simulink model "TuneControllers"  (R2020b)
settings: Solver=VariableStepAuto  StartTime=0.0  StopTime=10  RelTol=1e-3
undefined symbols (not defined in the file): Controller_Mode, DiscIntNeverNeededParam, Tests_Enum_SpectralTestSystem, ts_control
libraries: simulink x4
settings Model: DataDictionary=Dictionary.sldd  EnableAccessToBaseWorkspace=off  OrderedModelArguments=off  Creator=alons  LastModifiedBy=alons

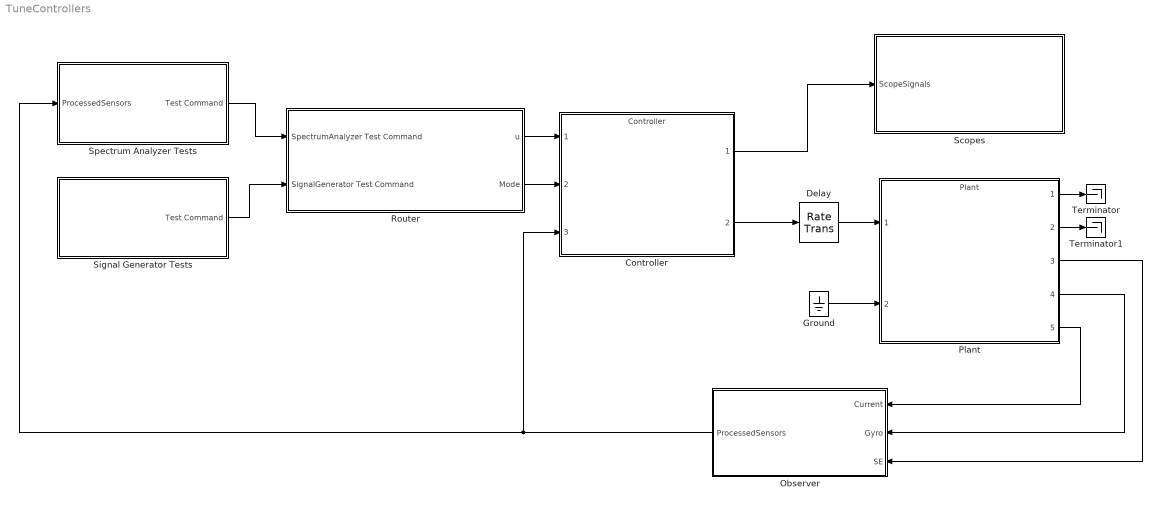
== system TuneControllers ==
  Controller : ModelReference  ModelNameDialog=Controller  SimulationMode=Normal  ModelReferenceVersion=1.79
  Delay : RateTransition  OutPortSampleTime=0
  Ground : Ground
  Observer : Subsystem  TreatAsAtomicUnit=on
  Plant : ModelReference  ModelNameDialog=Plant.slx  SimulationMode=Normal  ModelReferenceVersion=1.81  SimulationMode=Normal
  Router : Subsystem  TreatAsAtomicUnit=on
  Scopes : Subsystem
  Signal Generator Tests : Subsystem  TreatAsAtomicUnit=on
  Spectrum Analyzer Tests : Subsystem  TreatAsAtomicUnit=on
  Terminator : Terminator
  Terminator1 : Terminator
  wires:
  Delay/1 -> Plant/1
  Ground/1 -> Plant/2
  Observer/1(ProcessedSensors) -> Controller/3, Spectrum Analyzer Tests/1(ProcessedSensors)
  Signal Generator Tests/1(Test Command) -> Router/2(SignalGenerator Test Command)
  Spectrum Analyzer Tests/1(Test Command) -> Router/1(SpectrumAnalyzer Test Command)
  Router/1(u) -> Controller/1
  Router/2(Mode) -> Controller/2
  Plant/1 -> Terminator/1
  Controller/2 -> Delay/1
  Plant/5 -> Observer/1(Current)
  Plant/4 -> Observer/2(Gyro)
  Plant/3 -> Observer/3(SE)
  Plant/2 -> Terminator1/1
  Controller/1 -> Scopes/1(ScopeSignals)

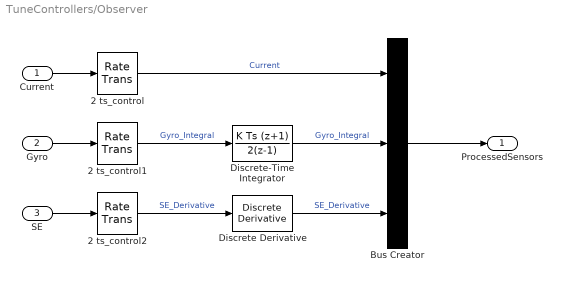
== system TuneControllers/Observer ==
  Current : Inport  SampleTime=ts_control
  Gyro : Inport  Port=2  SampleTime=ts_control
  SE : Inport  Port=3  SampleTime=ts_control
  2 ts_control : RateTransition  OutPortSampleTime=ts_control
  2 ts_control1 : RateTransition  OutPortSampleTime=ts_control
  2 ts_control2 : RateTransition  OutPortSampleTime=ts_control
  Bus Creator : BusCreator  Inputs=3  OutDataTypeStr=Bus: Processed_Sensors
  Discrete Derivative : simulink/Discrete/Discrete Derivative  gainval=1.0  ICPrevScaledInput=0.0  OutMin=[]  OutMax=[]  OutDataType=fixdt(1, 16)  OutScaling=2^-10  DoSatur=off
  Discrete-Time Integrator : DiscreteIntegrator  IntegratorMethod=Integration: Trapezoidal  SampleTime=-1  ICPrevOutput=DiscIntNeverNeededParam  ICPrevScaledInput=DiscIntNeverNeededParam
  ProcessedSensors : Outport  OutDataTypeStr=Bus: Processed_Sensors  SampleTime=ts_control
  wires:
  Bus Creator/1 -> ProcessedSensors/1
  Discrete Derivative/1 -> Bus Creator/3  "SE_Derivative"
  Discrete-Time Integrator/1 -> Bus Creator/2  "Gyro_Integral"
  2 ts_control1/1 -> Discrete-Time Integrator/1  "Gyro_Integral"
  Gyro/1 -> 2 ts_control1/1
  2 ts_control2/1 -> Discrete Derivative/1  "SE_Derivative"
  SE/1 -> 2 ts_control2/1
  Current/1 -> 2 ts_control/1
  2 ts_control/1 -> Bus Creator/1  "Current"

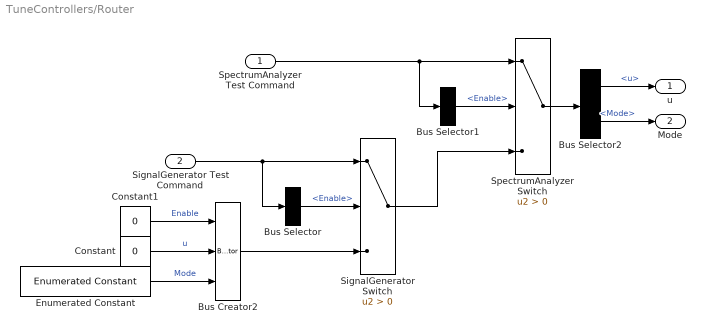
== system TuneControllers/Router ==
  SpectrumAnalyzer Test Command : Inport
  SignalGenerator Test Command : Inport  Port=2
  Bus Creator2 : BusCreator  Inputs=3
  Bus Selector : BusSelector  OutputSignals=Enable
  Bus Selector1 : BusSelector  OutputSignals=Enable
  Bus Selector2 : BusSelector  OutputSignals=u,Mode
  Constant : Constant  Value=0
  Constant1 : Constant  Value=0
  Enumerated Constant : simulink/Sources/Enumerated Constant  OutDataTypeStr=Enum: Controller_Mode  Value=Controller_Mode.Voltage  SampleTime=inf
  SignalGenerator Switch : Switch  Criteria=u2 > Threshold
  SpectrumAnalyzer Switch : Switch  Criteria=u2 > Threshold
  u : Outport
  Mode : Outport  Port=2
  wires:
  SignalGenerator Test Command/1 -> Bus Selector/1, SignalGenerator Switch/1
  Enumerated Constant/1 -> Bus Creator2/3  "Mode"
  Constant/1 -> Bus Creator2/2  "u"
  Bus Creator2/1 -> SignalGenerator Switch/3
  Bus Selector/1 -> SignalGenerator Switch/2  "<Enable>"
  SpectrumAnalyzer Test Command/1 -> Bus Selector1/1, SpectrumAnalyzer Switch/1
  Bus Selector1/1 -> SpectrumAnalyzer Switch/2  "<Enable>"
  SignalGenerator Switch/1 -> SpectrumAnalyzer Switch/3
  SpectrumAnalyzer Switch/1 -> Bus Selector2/1
  Constant1/1 -> Bus Creator2/1  "Enable"
  Bus Selector2/1 -> u/1  "<u>"
  Bus Selector2/2 -> Mode/1  "<Mode>"

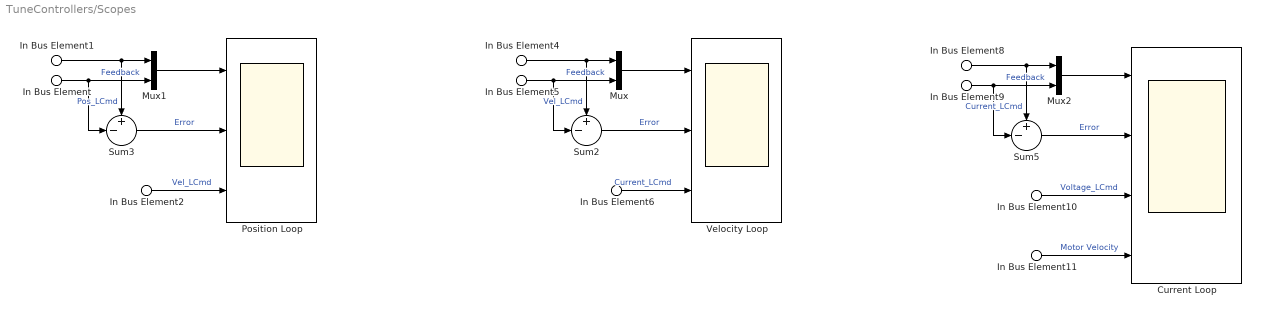
== system TuneControllers/Scopes ==
  In Bus Element : Inport  PortName=ScopeSignals  Element=Position.Gyro_Integral
  In Bus Element1 : Inport  PortName=ScopeSignals  Element=Position.Pos_LCmd
  In Bus Element2 : Inport  PortName=ScopeSignals  Element=Position.Vel_LCmd
  In Bus Element4 : Inport  PortName=ScopeSignals  Element=Velocity.Vel_LCmd
  In Bus Element5 : Inport  PortName=ScopeSignals  Element=Velocity.SE_Derivative
  In Bus Element6 : Inport  PortName=ScopeSignals  Element=Velocity.Current_LCmd
  In Bus Element8 : Inport  PortName=ScopeSignals  Element=Current.Current_LCmd
  In Bus Element9 : Inport  PortName=ScopeSignals  Element=Current.Current
  In Bus Element10 : Inport  PortName=ScopeSignals  Element=Current.Voltage_LCmd
  In Bus Element11 : Inport  PortName=ScopeSignals  Element=Current.SE_Derivative
  Current Loop : Scope  NumInputPorts=4
  Mux : Mux  Inputs=2
  Mux1 : Mux  Inputs=2
  Mux2 : Mux  Inputs=2
  Position Loop : Scope  NumInputPorts=3
  Sum2 : Sum  Inputs=+-|
  Sum3 : Sum  Inputs=+-|
  Sum5 : Sum  Inputs=+-|
  Velocity Loop : Scope  NumInputPorts=3
  wires:
  In Bus Element/1 -> Sum3/2, Mux1/2  "Feedback"
  In Bus Element8/1 -> Sum5/1, Mux2/1  "Current_LCmd"
  Sum5/1 -> Current Loop/2  "Error"
  In Bus Element10/1 -> Current Loop/3  "Voltage_LCmd"
  In Bus Element2/1 -> Position Loop/3  "Vel_LCmd"
  Mux2/1 -> Current Loop/1
  In Bus Element9/1 -> Sum5/2, Mux2/2  "Feedback"
  In Bus Element11/1 -> Current Loop/4  "Motor Velocity"
  In Bus Element5/1 -> Sum2/2, Mux/2  "Feedback"
  In Bus Element1/1 -> Sum3/1, Mux1/1  "Pos_LCmd"
  Mux/1 -> Velocity Loop/1
  In Bus Element6/1 -> Velocity Loop/3  "Current_LCmd"
  Mux1/1 -> Position Loop/1
  Sum3/1 -> Position Loop/2  "Error"
  In Bus Element4/1 -> Sum2/1, Mux/1  "Vel_LCmd"
  Sum2/1 -> Velocity Loop/2  "Error"

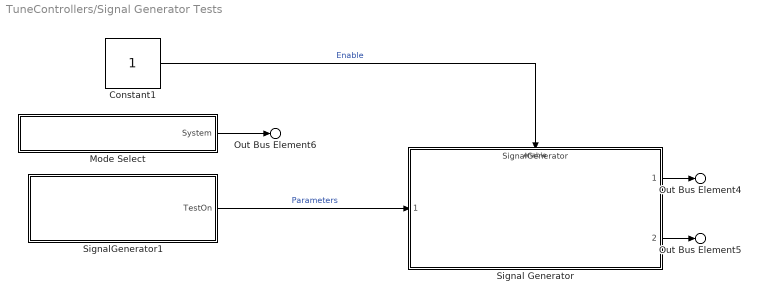
== system TuneControllers/Signal Generator Tests ==
  Constant1 : Constant  OutDataTypeStr=boolean
      settings: OpenFcn=|
      | if get_param(gcbh,'value')-48 set_param(gcbh,'value','0','backgroundcolor','red');
      | else set_param(gcbh,'value','1','backgroundcolor','green');
      | end
  Mode Select : Subsystem  mask(System Select){AxisMode=Velocity}
      mask prompts: AxisMode "Axis Mode for Test:"
      mask help: Specify the axis for test
      mask TypeOptions AxisMode: Voltage | Current | Velocity | Position
      mask Display:
      | Message = ['Selected Axis Mode: \n ' get_param(gcb,'AxisMode')];
      | disp(Message);
  Signal Generator : ModelReference  ModelNameDialog=SignalGenerator.slx  SimulationMode=Normal  ModelReferenceVersion=1.33  EnablePortName=Enable  EnablePortStatesWhenEnabling=reset
  SignalGenerator1 : Subsystem  mask(Signal Generator Parameters){TestType=Square wave, PeriodTime=2, Amplitude=20*pi/180, Bias=0, PulseWidth=20, NumberOfPeriods=100, ConstValue=1*pi/180}
      mask prompts: PeriodTime "Period time"; PulseWidth "Pulse width (%)"; NumberOfPeriods "Number of periods"
      mask help:
      | Comfy mask to create the input bus for Signal Generator.
      | If Constant is selected, only the ConstVal field is relevant.
      | (c) Alon Spinner 2021
      mask TypeOptions TestType: Square wave through zero | Square wave | Sine | Triangle | Pulse | Constant
      mask Callback TestType:
      | MaskObj=Simulink.Mask.get(gcb);
      | PeriodTimeObj= MaskObj.getParameter('PeriodTime');
      | AmplitudeObj= MaskObj.getParameter('Amplitude');
      | BiasObj= MaskObj.getParameter('Bias');
      | PulseWidthObj= MaskObj.getParameter('PulseWidth');
      | NumberOfPeriodsObj= MaskObj.getParameter('NumberOfPeriods');
      | ConstValueObj= MaskObj.getParameter('ConstValue');
      | 
      | switch get_param(gcb,'TestType')
      | 
      |     case {'Square wave through zero','Square wave','Sine','Triangle'}
      |         PeriodTimeObj.Visible='on';
      |         AmplitudeObj.Visible='on';
      |         BiasObj.Visible='on';
      |         PulseWidthObj.Visible='off';
      |         NumberOfPeriodsObj.Visible='on';
      |         ConstValueObj.Visible='off';
      |     case 'Pulse'
      |         PeriodTimeObj.Visible='on';
      |         AmplitudeObj.Visible='on';
      |         BiasObj.Visible='on';
      |         PulseWidthObj.Visible='on';
      |         NumberOfPeriodsObj.Visible='on';
      |         ConstValueObj.Visible='off';
      |     case 'Constant'
      |         PeriodTimeObj.Visible='off';
      |         AmplitudeObj.Visible='off';
      |         BiasObj.Visible='off';
      |         PulseWidthObj.Visible='off';
      |         NumberOfPeriodsObj.Visible='off';
      |         ConstValueObj.Visible='on';
      | end
      mask Display:
      | disp('Signal Generator Parameters\n----------------------------\n\n\n\n')
      | 
      | switch TestType
      |     case 1
      |         disp('\n\nTest Type:\nSquare wave through zero')
      |     case 2
      |         disp('\n\nTest Type:\nSquare wave')
      |     case 3
      |         disp('\n\nTest Type:\nSine wave')
      |     case 4
      |         disp('\n\nTest Type:\nTriangle wave')
      |     case 5
      |         disp('\n\nTest Type:\nPulse')
      |     case 6
      |         disp('\n\nTest Type:\nConstant')
      | end
  Out Bus Element4 : Outport  PortName=Test Command  Element=Enable
  Out Bus Element5 : Outport  PortName=Test Command  Element=u
  Out Bus Element6 : Outport  PortName=Test Command  Element=Mode
  wires:
  Constant1/1 -> Signal Generator/Enable  "Enable"
  SignalGenerator1/1(TestOn) -> Signal Generator/1  "Parameters"
  Mode Select/1(System) -> Out Bus Element6/1
  Signal Generator/2 -> Out Bus Element5/1
  Signal Generator/1 -> Out Bus Element4/1

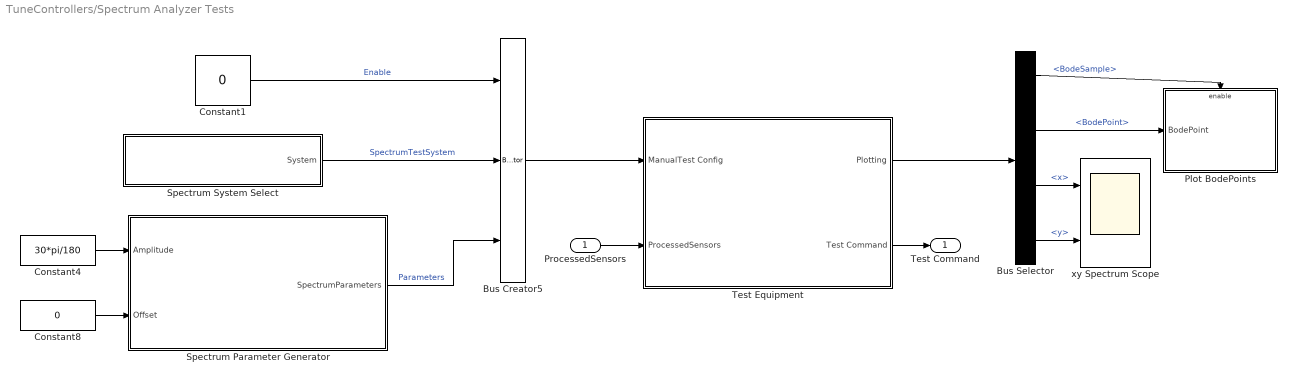
== system TuneControllers/Spectrum Analyzer Tests ==
  ProcessedSensors : Inport
  Bus Creator5 : BusCreator  Inputs=3
  Bus Selector : BusSelector  OutputSignals=BodeSample,BodePoint,x,y
  Constant1 : Constant  Value=0  OutDataTypeStr=boolean
      settings: OpenFcn=|
      | if get_param(gcbh,'value')-48 set_param(gcbh,'value','0','backgroundcolor','red');
      | else set_param(gcbh,'value','1','backgroundcolor','green');
      | end
  Constant4 : Constant  Value=30*pi/180  OutDataTypeStr=Inherit: Inherit via back propagation
  Constant8 : Constant  Value=0  OutDataTypeStr=Inherit: Inherit via back propagation
  Plot BodePoints : Subsystem
  Spectrum Parameter Generator : Subsystem  mask{PhaseIn=0, Start_Frequency=1, Stop_Frequency=500, Min_PeriodsPerSine=5, Min_PointsPerSine=150, LinearOrLog=Logarithmic, Linear_Step_Frequency=0.1, Logarithmic_NumOfPoints=250, OLCL=CL}
      mask prompts: PhaseIn "Phase In [rad]"; Start_Frequency "Start Frequency [Hz]"; Stop_Frequency "Stop Frequency [Hz]"; Min_PeriodsPerSine "Minimal Number of periods per frequency"; Min_PointsPerSine "Minimal Number of sampled points per frequency"; LinearOrLog "Frequency axis type"; Linear_Step_Frequency "Step Frequency [Hz] (for linear test type)"; Logarithmic_NumOfPoints "Number of points (for logarithmic test type)"; OLCL "Measurement Type"
      mask init:
      | switch LinearOrLog
      |     case 1
      |         f = Start_Frequency:Linear_Step_Frequency:Stop_Frequency;
      |         n = length(f);
      |     case 2
      |         n = 1:Logarithmic_NumOfPoints;
      |         f = 10.^((log10(Stop_Frequency) - log10(Start_Frequency))/Logarithmic_NumOfPoints*n + log10(Start_Frequency));
      | end
      | %%%%%%%%%%%%%%%%%%%%%%%%%%%%
      | ts=1/1024; %assumption
      | T_min=Min_PointsPerSine*ts; %scalar
      | T_minPeriodsPerSine=Min_PeriodsPerSine*(1./f); %vector
      | T=sum(max(T_minPeriodsPerSine,T_min));
      | 
      | y = T/60; 
      | h = floor(y/60); %[hours]
      | m = floor(((y/60)-h)*60); %[min]
      | s = round((y-floor(y))*60); %[sec]
      mask TypeOptions LinearOrLog: Linear | Logarithmic
      mask Callback LinearOrLog:
      | MaskObj = Simulink.Mask.get(gcb);
      | Linear_Step_Frequency_Obj= MaskObj.getParameter('Linear_Step_Frequency');
      | Logarithmic_NumOfPoints_Obj= MaskObj.getParameter('Logarithmic_NumOfPoints');
      | 
      | LinearOrLog = get_param(gcb,'LinearOrLog');
      | switch LinearOrLog
      |     case 'Linear'
      |     Linear_Step_Frequency_Obj.Visible='on';
      |     Logarithmic_NumOfPoints_Obj.Visible='off';
      |     case 'Logarithmic'
      |     Linear_Step_Frequency_Obj.Visible='off';
      |     Logarithmic_NumOfPoints_Obj.Visible='on';
      | end
      mask TypeOptions OLCL: OL | CL
      mask DialogControl Container3 Prompt: Test Type
      mask Display:
      | str = sprintf(['-----------------\n'...
      |     'SPECTRUM\nParameter\nGenerator\n',...
      |     '------------------\n',...
      |     'Estimated test time:\n',...
      |     '%02d:%02d:%02d\n[hh:mm:ss]'],h,m,s);
      | disp(str)
  Spectrum System Select : Subsystem  mask(System Select){SpectralTestSystem=SE_Velocity_CL}
      mask help: Specify the axis for test
      mask TypeOptions SpectralTestSystem: NoSpectralTest | Current_Plant | Current_CL | SE_Velocity_Plant | SE_Velocity_CL | Gyro_Position_Plant | Gyro_Position_CL
      mask Display:
      | if ~strcmpi(get_param(gcb,'SpectralTestSystem'),'NoSpectralTest'),
      |     set_param(gcb,'BackgroundColor','Green');
      |     Message = [' *** ACTIVE *** \n Selected Axis: \n ' get_param(gcb,'SpectralTestSystem')];
      | else
      |     set_param(gcb,'BackgroundColor','Red');
      |      Message = [' *** deactivated ***'];
      | end
      | 
      | disp(Message);
  Test Equipment : Subsystem  TreatAsAtomicUnit=on
  xy Spectrum Scope : Scope  NumInputPorts=2
  Test Command : Outport
  wires:
  Test Equipment/2(Test Command) -> Test Command/1
  Bus Creator5/1 -> Test Equipment/1(ManualTest Config)
  Constant1/1 -> Bus Creator5/1  "Enable"
  Constant4/1 -> Spectrum Parameter Generator/1(Amplitude)
  Constant8/1 -> Spectrum Parameter Generator/2(Offset)
  Spectrum System Select/1(System) -> Bus Creator5/2  "SpectrumTestSystem"
  Bus Selector/3 -> xy Spectrum Scope/1  "<x>"
  Bus Selector/1 -> Plot BodePoints/Enable  "<BodeSample>"
  Bus Selector/2 -> Plot BodePoints/1(BodePoint)  "<BodePoint>"
  Bus Selector/4 -> xy Spectrum Scope/2  "<y>"
  Test Equipment/1(Plotting) -> Bus Selector/1
  Spectrum Parameter Generator/1(SpectrumParameters) -> Bus Creator5/3  "Parameters"
  ProcessedSensors/1 -> Test Equipment/2(ProcessedSensors)

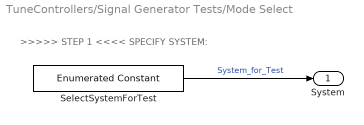
== system TuneControllers/Signal Generator Tests/Mode Select ==
  note: >>>>> STEP 1 <<<< SPECIFY SYSTEM:
  SelectSystemForTest : simulink/Sources/Enumerated Constant  OutDataTypeStr=Enum: Controller_Mode  Value=Controller_Mode(AxisMode)  SampleTime=inf
  System : Outport
  wires:
  SelectSystemForTest/1 -> System/1  "System_for_Test"

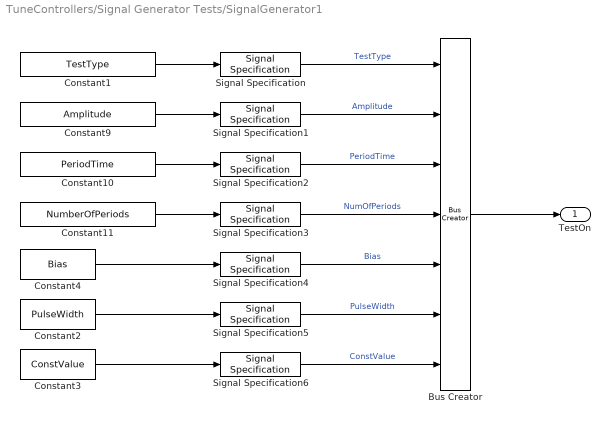
== system TuneControllers/Signal Generator Tests/SignalGenerator1 ==
  Bus Creator : BusCreator  Inputs=7  OutDataTypeStr=Bus: Tests_SignalGenerator_Parameters  NonVirtualBus=on
  Constant1 : Constant  Value=TestType  OutDataTypeStr=Inherit: Inherit via back propagation
  Constant10 : Constant  Value=PeriodTime  OutDataTypeStr=Inherit: Inherit via back propagation
  Constant11 : Constant  Value=NumberOfPeriods  OutDataTypeStr=Inherit: Inherit via back propagation
  Constant2 : Constant  Value=PulseWidth  OutDataTypeStr=Inherit: Inherit via back propagation
  Constant3 : Constant  Value=ConstValue  OutDataTypeStr=Inherit: Inherit via back propagation
  Constant4 : Constant  Value=Bias  OutDataTypeStr=Inherit: Inherit via back propagation
  Constant9 : Constant  Value=Amplitude  OutDataTypeStr=Inherit: Inherit via back propagation
  Signal Specification : SignalSpecification  OutDataTypeStr=int8
  Signal Specification{1..6} (6 alike) : SignalSpecification  OutDataTypeStr=double
  TestOn : Outport  OutDataTypeStr=Bus: Tests_SignalGenerator_Parameters  OutputWhenDisabled=reset  InitialOutput=0
  wires:
  Constant1/1 -> Signal Specification/1
  Constant9/1 -> Signal Specification1/1
  Constant4/1 -> Signal Specification4/1
  Constant11/1 -> Signal Specification3/1
  Constant10/1 -> Signal Specification2/1
  Bus Creator/1 -> TestOn/1
  Constant2/1 -> Signal Specification5/1
  Signal Specification/1 -> Bus Creator/1  "TestType"
  Signal Specification1/1 -> Bus Creator/2  "Amplitude"
  Signal Specification2/1 -> Bus Creator/3  "PeriodTime"
  Signal Specification3/1 -> Bus Creator/4  "NumOfPeriods"
  Signal Specification4/1 -> Bus Creator/5  "Bias"
  Signal Specification5/1 -> Bus Creator/6  "PulseWidth"
  Signal Specification6/1 -> Bus Creator/7  "ConstValue"
  Constant3/1 -> Signal Specification6/1

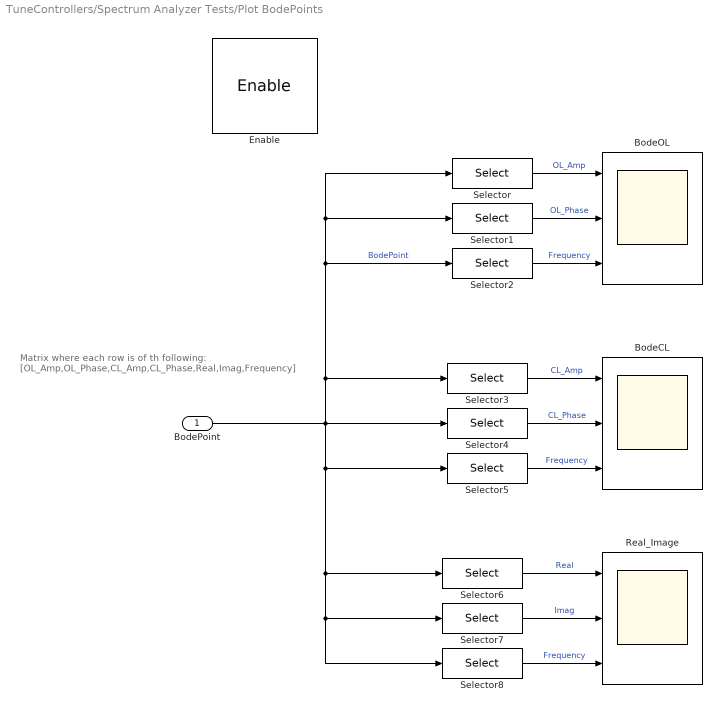
== system TuneControllers/Spectrum Analyzer Tests/Plot BodePoints ==
  note: Matrix where each row is of th following:
      | [OL_Amp,OL_Phase,CL_Amp,CL_Phase,Real,Imag,Frequency]
  BodePoint : Inport
  Enable : EnablePort  StatesWhenEnabling=reset
  BodeCL : Scope  NumInputPorts=3
  BodeOL : Scope  NumInputPorts=3
  Real_Image : Scope  NumInputPorts=3
  Selector : Selector  NumberOfDimensions=2  InputPortWidth=3  IndexOptions=Select all,Index vector (dialog)  Indices=1,1  OutputSizes=1,1
  Selector1 : Selector  NumberOfDimensions=2  InputPortWidth=3  IndexOptions=Select all,Index vector (dialog)  Indices=1,2  OutputSizes=1,1
  Selector2 : Selector  NumberOfDimensions=2  InputPortWidth=3  IndexOptions=Select all,Index vector (dialog)  Indices=1,7  OutputSizes=1,1
  Selector3 : Selector  NumberOfDimensions=2  InputPortWidth=3  IndexOptions=Select all,Index vector (dialog)  Indices=1,3  OutputSizes=1,1
  Selector4 : Selector  NumberOfDimensions=2  InputPortWidth=3  IndexOptions=Select all,Index vector (dialog)  Indices=1,4  OutputSizes=1,1
  Selector5 : Selector  NumberOfDimensions=2  InputPortWidth=3  IndexOptions=Select all,Index vector (dialog)  Indices=1,7  OutputSizes=1,1
  Selector6 : Selector  NumberOfDimensions=2  InputPortWidth=3  IndexOptions=Select all,Index vector (dialog)  Indices=1,5  OutputSizes=1,1
  Selector7 : Selector  NumberOfDimensions=2  InputPortWidth=3  IndexOptions=Select all,Index vector (dialog)  Indices=1,6  OutputSizes=1,1
  Selector8 : Selector  NumberOfDimensions=2  InputPortWidth=3  IndexOptions=Select all,Index vector (dialog)  Indices=1,7  OutputSizes=1,1
  wires:
  BodePoint/1 -> Selector/1, Selector1/1, Selector2/1, Selector3/1, Selector4/1, Selector5/1, Selector6/1, Selector7/1, Selector8/1  "BodePoint"
  Selector8/1 -> Real_Image/3  "Frequency"
  Selector7/1 -> Real_Image/2  "Imag"
  Selector6/1 -> Real_Image/1  "Real"
  Selector5/1 -> BodeCL/3  "Frequency"
  Selector4/1 -> BodeCL/2  "CL_Phase"
  Selector3/1 -> BodeCL/1  "CL_Amp"
  Selector2/1 -> BodeOL/3  "Frequency"
  Selector1/1 -> BodeOL/2  "OL_Phase"
  Selector/1 -> BodeOL/1  "OL_Amp"

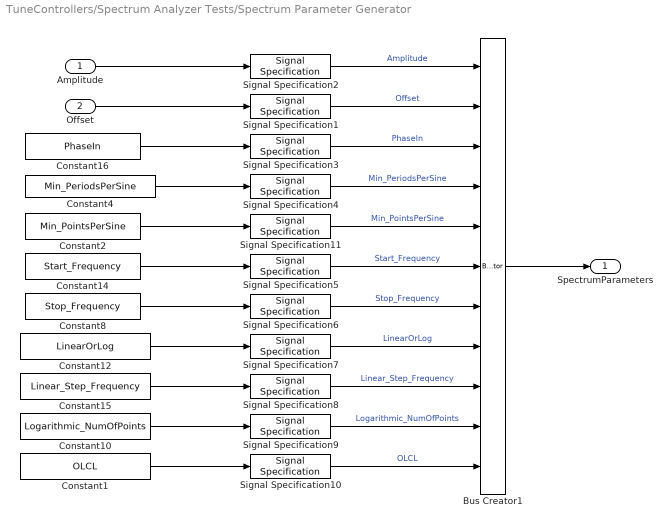
== system TuneControllers/Spectrum Analyzer Tests/Spectrum Parameter Generator ==
  Amplitude : Inport
  Offset : Inport  Port=2
  Bus Creator1 : BusCreator  Inputs=11  OutDataTypeStr=Bus: Tests_SpectrumAnalyzer_Parameters  NonVirtualBus=on
  Constant1 : Constant  Value=OLCL  OutDataTypeStr=Inherit: Inherit via back propagation
  Constant10 : Constant  Value=Logarithmic_NumOfPoints  OutDataTypeStr=Inherit: Inherit via back propagation
  Constant12 : Constant  Value=LinearOrLog  OutDataTypeStr=Inherit: Inherit via back propagation
  Constant14 : Constant  Value=Start_Frequency  OutDataTypeStr=Inherit: Inherit via back propagation
  Constant15 : Constant  Value=Linear_Step_Frequency  OutDataTypeStr=Inherit: Inherit via back propagation
  Constant16 : Constant  Value=PhaseIn  OutDataTypeStr=Inherit: Inherit via back propagation
  Constant2 : Constant  Value=Min_PointsPerSine  OutDataTypeStr=Inherit: Inherit via back propagation
  Constant4 : Constant  Value=Min_PeriodsPerSine  OutDataTypeStr=Inherit: Inherit via back propagation
  Constant8 : Constant  Value=Stop_Frequency  OutDataTypeStr=Inherit: Inherit via back propagation
  Signal Specification{1..6,8..9,11} (9 alike) : SignalSpecification  OutDataTypeStr=double
  Signal Specification10 : SignalSpecification  OutDataTypeStr=int8
  Signal Specification7 : SignalSpecification  OutDataTypeStr=int8
  SpectrumParameters : Outport  OutDataTypeStr=Bus: Tests_SpectrumAnalyzer_Parameters
  wires:
  Signal Specification11/1 -> Bus Creator1/5  "Min_PointsPerSine"
  Constant2/1 -> Signal Specification11/1
  Constant10/1 -> Signal Specification9/1
  Constant14/1 -> Signal Specification5/1
  Constant8/1 -> Signal Specification6/1
  Constant15/1 -> Signal Specification8/1
  Offset/1 -> Signal Specification1/1
  Amplitude/1 -> Signal Specification2/1
  Constant16/1 -> Signal Specification3/1
  Constant4/1 -> Signal Specification4/1
  Signal Specification2/1 -> Bus Creator1/1  "Amplitude"
  Signal Specification1/1 -> Bus Creator1/2  "Offset"
  Bus Creator1/1 -> SpectrumParameters/1
  Constant1/1 -> Signal Specification10/1
  Constant12/1 -> Signal Specification7/1
  Signal Specification3/1 -> Bus Creator1/3  "PhaseIn"
  Signal Specification4/1 -> Bus Creator1/4  "Min_PeriodsPerSine"
  Signal Specification5/1 -> Bus Creator1/6  "Start_Frequency"
  Signal Specification6/1 -> Bus Creator1/7  "Stop_Frequency"
  Signal Specification7/1 -> Bus Creator1/8  "LinearOrLog"
  Signal Specification8/1 -> Bus Creator1/9  "Linear_Step_Frequency"
  Signal Specification9/1 -> Bus Creator1/10  "Logarithmic_NumOfPoints"
  Signal Specification10/1 -> Bus Creator1/11  "OLCL"

== system TuneControllers/Spectrum Analyzer Tests/Spectrum System Select ==
  note: >>>>> STEP 1 <<<< SPECIFY SYSTEM:
  SelectSystemForTest : simulink/Sources/Enumerated Constant  OutDataTypeStr=Enum: Tests_Enum_SpectralTestSystem  Value=Tests_Enum_SpectralTestSystem(SpectralTestSystem)  SampleTime=inf
  System : Outport
  wires:
  SelectSystemForTest/1 -> System/1

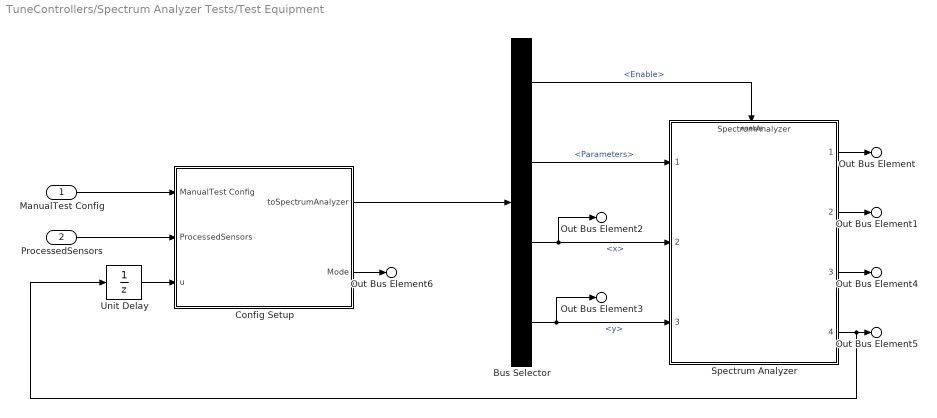
== system TuneControllers/Spectrum Analyzer Tests/Test Equipment ==
  ManualTest Config : Inport
  ProcessedSensors : Inport  Port=2
  Bus Selector : BusSelector  OutputSignals=Enable,Parameters,x,y
  Config Setup : Subsystem  TreatAsAtomicUnit=on
  Spectrum Analyzer : ModelReference  ModelNameDialog=SpectrumAnalyzer.slx  SimulationMode=Normal  ModelReferenceVersion=2.53  EnablePortName=Enable  EnablePortStatesWhenEnabling=reset
  Unit Delay : UnitDelay  SampleTime=-1  HasFrameUpgradeWarning=on
  Out Bus Element : Outport  PortName=Plotting  Element=BodeSample
  Out Bus Element1 : Outport  PortName=Plotting  Element=BodePoint
  Out Bus Element2 : Outport  PortName=Plotting  Element=x
  Out Bus Element3 : Outport  PortName=Plotting  Element=y
  Out Bus Element4 : Outport  Port=2  PortName=Test Command  Element=Enable
  Out Bus Element5 : Outport  Port=2  PortName=Test Command  Element=u
  Out Bus Element6 : Outport  Port=2  PortName=Test Command  Element=Mode
  wires:
  ManualTest Config/1 -> Config Setup/1(ManualTest Config)
  Spectrum Analyzer/1 -> Out Bus Element/1
  Spectrum Analyzer/2 -> Out Bus Element1/1
  Bus Selector/4 -> Spectrum Analyzer/3, Out Bus Element3/1  "<y>"
  Config Setup/1(toSpectrumAnalyzer) -> Bus Selector/1
  Bus Selector/2 -> Spectrum Analyzer/1  "<Parameters>"
  Bus Selector/1 -> Spectrum Analyzer/Enable  "<Enable>"
  Bus Selector/3 -> Spectrum Analyzer/2, Out Bus Element2/1  "<x>"
  Spectrum Analyzer/3 -> Out Bus Element4/1
  Spectrum Analyzer/4 -> Unit Delay/1, Out Bus Element5/1
  Config Setup/2(Mode) -> Out Bus Element6/1
  ProcessedSensors/1 -> Config Setup/2(ProcessedSensors)
  Unit Delay/1 -> Config Setup/3(u)

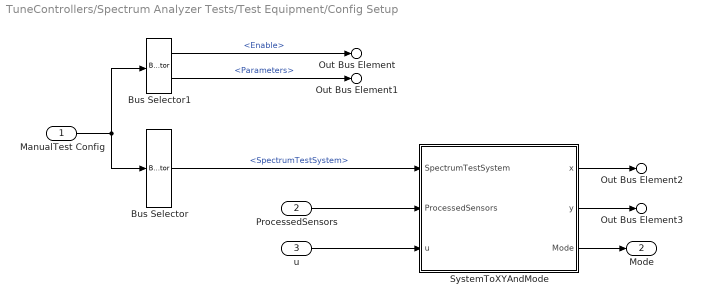
== system TuneControllers/Spectrum Analyzer Tests/Test Equipment/Config Setup ==
  ManualTest Config : Inport
  ProcessedSensors : Inport  Port=2
  u : Inport  Port=3
  Bus Selector : BusSelector  OutputSignals=SpectrumTestSystem
  Bus Selector1 : BusSelector  OutputSignals=Enable,Parameters
  SystemToXYAndMode : MATLAB Function  TreatAsAtomicUnit=on
  Out Bus Element : Outport  PortName=toSpectrumAnalyzer  Element=Enable
  Out Bus Element1 : Outport  PortName=toSpectrumAnalyzer  Element=Parameters
  Out Bus Element2 : Outport  PortName=toSpectrumAnalyzer  Element=x
  Out Bus Element3 : Outport  PortName=toSpectrumAnalyzer  Element=y
  Mode : Outport  Port=2
  wires:
  SystemToXYAndMode/3(Mode) -> Mode/1
  SystemToXYAndMode/1(x) -> Out Bus Element2/1
  SystemToXYAndMode/2(y) -> Out Bus Element3/1
  Bus Selector1/1 -> Out Bus Element/1  "<Enable>"
  Bus Selector1/2 -> Out Bus Element1/1  "<Parameters>"
  ManualTest Config/1 -> Bus Selector1/1, Bus Selector/1
  Bus Selector/1 -> SystemToXYAndMode/1(SpectrumTestSystem)  "<SpectrumTestSystem>"
  ProcessedSensors/1 -> SystemToXYAndMode/2(ProcessedSensors)
  u/1 -> SystemToXYAndMode/3(u)

== matlab function TuneControllers/Spectrum Analyzer Tests/Test Equipment/Config Setup/SystemToXYAndMode ==
  data: SpectrumTestSystem input; ProcessedSensors input; u input; x output size=1; y output size=1; Mode output
function [x,y,Mode]=SystemToXYAndMode(SpectrumTestSystem,ProcessedSensors,u)%#codegen
x=u;
y=0;
Mode=Controller_Mode.Voltage;

switch SpectrumTestSystem
    case Tests_Enum_SpectralTestSystem.Current_Plant
        Mode=Controller_Mode.Voltage;
        y=ProcessedSensors.Current;
        
    case Tests_Enum_SpectralTestSystem.Current_CL
        Mode=Controller_Mode.Current;
        y=ProcessedSensors.Current;
    
    case Tests_Enum_SpectralTestSystem.SE_Velocity_Plant
        Mode=Controller_Mode.Current;
        y=ProcessedSensors.SE_Derivative;
        
    case Tests_Enum_SpectralTestSystem.SE_Velocity_CL
        Mode=Controller_Mode.Velocity;
        y=ProcessedSensors.SE_Derivative;
        
    case Tests_Enum_SpectralTestSystem.Gyro_Position_Plant
        Mode=Controller_Mode.Velocity;
        y=ProcessedSensors.Gyro_Integral;
        
    case Tests_Enum_SpectralTestSystem.Gyro_Position_CL
        Mode=Controller_Mode.Position;
        y=ProcessedSensors.Gyro_Integral;
end
